simulink model "chap2_8sim"  (Simulink 3.00)
settings: Solver=ode45  StartTime=0.0  StopTime=5  RelTol=1e-3
settings Model: LastModifiedBy=liu

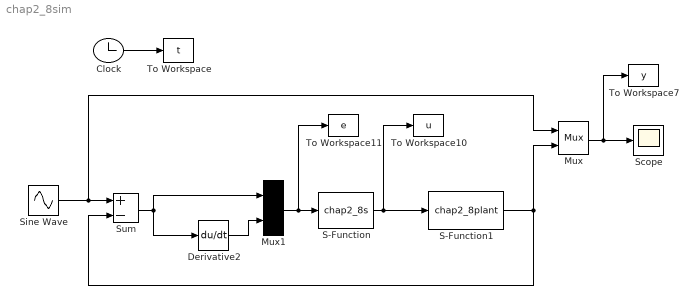
== system chap2_8sim ==
  Clock : Clock
  Derivative2 : Derivative
  Mux : Mux  Inputs=2
      settings: DisplayOption=none
  Mux1 : Mux  Inputs=2
      settings: DisplayOption=none
  S-Function : S-Function  FunctionName=chap2_8s  PortCounts=[]  SFunctionModules=''
  S-Function1 : S-Function  FunctionName=chap2_8plant  PortCounts=[]  SFunctionModules=''
  Scope : Scope
      settings: TimeRange=3  YMin=6.77626e-020  YMax=0.0009  SaveToWorkspace=off  SaveName=ScopeData  MaxRows=500000
  Sine Wave : Sin  Amplitude=1  Frequency=2*pi  Phase=0  SampleTime=0
  Sum : Sum  Inputs=+-  SaturateOnIntegerOverflow=on
  To Workspace : ToWorkspace  VariableName=t  SampleTime=-1  SaveFormat=Matrix
  To Workspace10 : ToWorkspace  VariableName=u  SampleTime=-1  SaveFormat=Matrix
  To Workspace11 : ToWorkspace  VariableName=e  SampleTime=-1  SaveFormat=Matrix
  To Workspace7 : ToWorkspace  VariableName=y  SampleTime=-1  SaveFormat=Matrix
  wires:
  Sine Wave/1 -> Sum/1, Mux/1
  S-Function/1 -> To Workspace10/1, S-Function1/1
  Derivative2/1 -> Mux1/2
  Sum/1 -> Derivative2/1, Mux1/1
  Mux1/1 -> S-Function/1, To Workspace11/1
  Clock/1 -> To Workspace/1
  Mux/1 -> Scope/1, To Workspace7/1
  S-Function1/1 -> Mux/2, Sum/2
